simulink model "catvehicle_hoffmannFollower"  (R2016a)
settings: Solver=FixedStepAuto  StartTime=0.0  StopTime=inf  FixedStep=0.05  RelTol=1e-3
undefined symbols (not defined in the file or in its folder): Angular, Linear, Pose
libraries: robotlib x5, aerolibtransform2 x2
settings Model: Creator=sprinkle  LastModifiedBy=sprinkle
settings DataIOCC: LimitDataPoints=on
settings OptimizationCC: OptimizeModelRefInitCode=on  LifeSpan=Inf  MaxStackSize=64
settings DebuggingCC: AllowSymbolicDim=off
settings HardwareCC: ProdBitPerPointer=32  ProdLargestAtomicFloat=None  ProdIntDivRoundTo=Undefined  ProdEndianess=Unspecified  ProdWordSize=32  ProdHWDeviceType=Generic->Unspecified (assume 32-bit Generic)
settings ModelReferenceCC: PropagateSignalLabelsOutOfModel=off
settings RTWCC: SystemTargetFile=ert.tlc  HardwareBoard=Robot Operating System (ROS)  TemplateMakefile=ert_default_tmf  GenerateReport=on  Toolchain=Catkin  BuildConfiguration=Faster Runs  IncludeHyperlinkInReport=on  LaunchReport=on  TargetLang=C++  GenerateTraceInfo=on  GenerateTraceReport=on  GenerateTraceReportSl=on  GenerateTraceReportSf=on  GenerateTraceReportEml=on
settings CodeAppCC: ForceParamTrailComments=on  IgnoreCustomStorageClasses=off  OperatorAnnotations=on  SimulinkDataObjDesc=on  SFDataObjDesc=on  MATLABFcnDesc=on  InsertBlockDesc=on  MATLABSourceComments=on

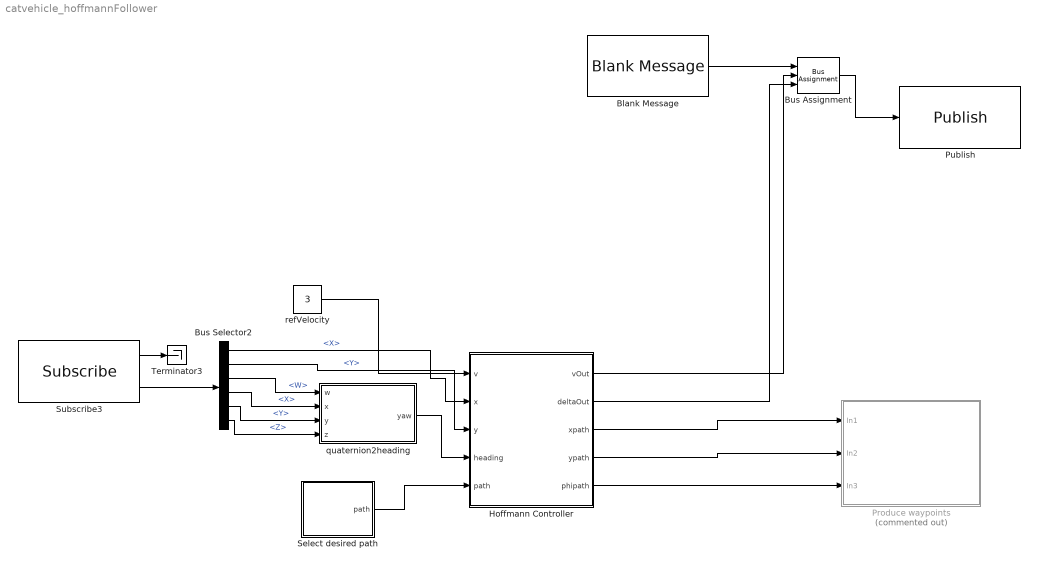
== system catvehicle_hoffmannFollower ==
  Blank Message : robotlib/Blank Message  SourceLibraryInfo=This block requires Robotics System Toolbox  messageType=geometry_msgs/Twist  SampleTime=inf
  Bus Assignment : BusAssignment  AssignedSignals=Linear.X,Angular.Z
  Bus Selector2 : BusSelector  OutputSignals=Pose.Pose.Position.X,Pose.Pose.Position.Y,Pose.Pose.Orientation.W,Pose.Pose.Orientation.X,Pose.Pose.Orientation.Y,Pose.Pose.Orientation.Z
  Hoffmann Controller : Subsystem
  Produce waypoints : Subsystem  Commented=on
  Publish : robotlib/Publish  SourceLibraryInfo=This block requires Robotics System Toolbox  topicSource=Specify your own  topic=/catvehicle/cmd_vel  messageType=geometry_msgs/Twist  messageQueueLength=1
  Select desired path : Subsystem
  Subscribe3 : robotlib/Subscribe  SourceLibraryInfo=This block requires Robotics System Toolbox  topicSource=Specify your own  topic=/catvehicle/odom  messageType=nav_msgs/Odometry  sampleTime=-1  messageQueueLength=1
  Terminator3 : Terminator
  quaternion2heading : Subsystem
  refVelocity : Constant  Value=3
  wires:
  Blank Message/1 -> Bus Assignment/1
  Bus Assignment/1 -> Publish/1
  Subscribe3/1 -> Terminator3/1
  Subscribe3/2 -> Bus Selector2/1
  refVelocity/1 -> Hoffmann Controller/1(v)
  Bus Selector2/1 -> Hoffmann Controller/2(x)  "<X>"
  Bus Selector2/2 -> Hoffmann Controller/3(y)  "<Y>"
  Hoffmann Controller/2(deltaOut) -> Bus Assignment/3
  Select desired path/1(path) -> Hoffmann Controller/5(path)
  quaternion2heading/1(yaw) -> Hoffmann Controller/4(heading)
  Bus Selector2/3 -> quaternion2heading/1(w)  "<W>"
  Bus Selector2/4 -> quaternion2heading/2(x)  "<X>"
  Bus Selector2/5 -> quaternion2heading/3(y)  "<Y>"
  Bus Selector2/6 -> quaternion2heading/4(z)  "<Z>"
  Hoffmann Controller/1(vOut) -> Bus Assignment/2
  Hoffmann Controller/3(xpath) -> Produce waypoints/1(In1)
  Hoffmann Controller/4(ypath) -> Produce waypoints/2(In2)
  Hoffmann Controller/5(phipath) -> Produce waypoints/3(In3)

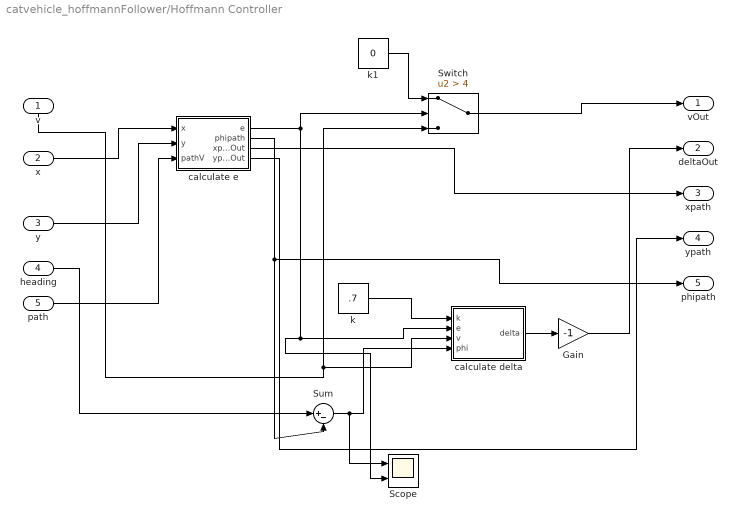
== system catvehicle_hoffmannFollower/Hoffmann Controller ==
  v : Inport
  x : Inport  Port=2
  y : Inport  Port=3
  heading : Inport  Port=4
  path : Inport  Port=5
  Gain : Gain  Gain=-1
  Scope : Scope  NumInputPorts=2
  Sum : Sum  Inputs=|+-
  Switch : Switch  Criteria=u2 > Threshold  Threshold=4
  calculate delta : MATLAB Function  TreatAsAtomicUnit=on
  calculate e : MATLAB Function  TreatAsAtomicUnit=on
  k : Constant  Value=.7
  k1 : Constant  Value=0
  vOut : Outport
  deltaOut : Outport  Port=2
  xpath : Outport  Port=3
  ypath : Outport  Port=4
  phipath : Outport  Port=5
  wires:
  v/1 -> Switch/3, calculate delta/3(v)
  path/1 -> calculate e/3(pathV)
  x/1 -> calculate e/1(x)
  y/1 -> calculate e/2(y)
  calculate e/2(phipath) -> phipath/1, Sum/2
  calculate e/1(e) -> Switch/2, Scope/2, calculate delta/2(e)
  Sum/1 -> Scope/1, calculate delta/4(phi)
  k/1 -> calculate delta/1(k)
  calculate e/3(xpathOut) -> xpath/1
  calculate e/4(ypathOut) -> ypath/1
  Switch/1 -> vOut/1
  k1/1 -> Switch/1
  heading/1 -> Sum/1
  calculate delta/1(delta) -> Gain/1
  Gain/1 -> deltaOut/1

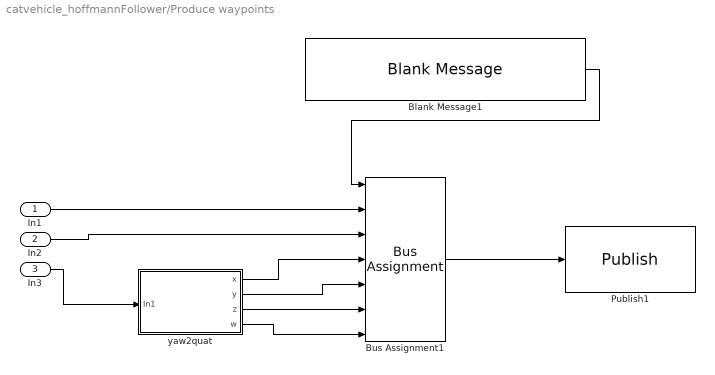
== system catvehicle_hoffmannFollower/Produce waypoints ==
  In1 : Inport
  In2 : Inport  Port=2
  In3 : Inport  Port=3
  Blank Message1 : robotlib/Blank Message  SourceLibraryInfo=This block requires Robotics System Toolbox  messageType=visualization_msgs/InteractiveMarkerPose  SampleTime=inf
  Bus Assignment1 : BusAssignment  AssignedSignals=Pose.Position.X,Pose.Position.Y,Pose.Orientation.X,Pose.Orientation.Y,Pose.Orientation.Z,Pose.Orientation.W
  Publish1 : robotlib/Publish  SourceLibraryInfo=This block requires Robotics System Toolbox  topicSource=Specify your own  topic=/catvehicle/waypoint  messageType=visualization_msgs/InteractiveMarkerPose  messageQueueLength=1
  yaw2quat : Subsystem
  wires:
  Blank Message1/1 -> Bus Assignment1/1
  Bus Assignment1/1 -> Publish1/1
  In1/1 -> Bus Assignment1/2
  In2/1 -> Bus Assignment1/3
  In3/1 -> yaw2quat/1(In1)
  yaw2quat/1(x) -> Bus Assignment1/4
  yaw2quat/2(y) -> Bus Assignment1/5
  yaw2quat/3(z) -> Bus Assignment1/6
  yaw2quat/4(w) -> Bus Assignment1/7

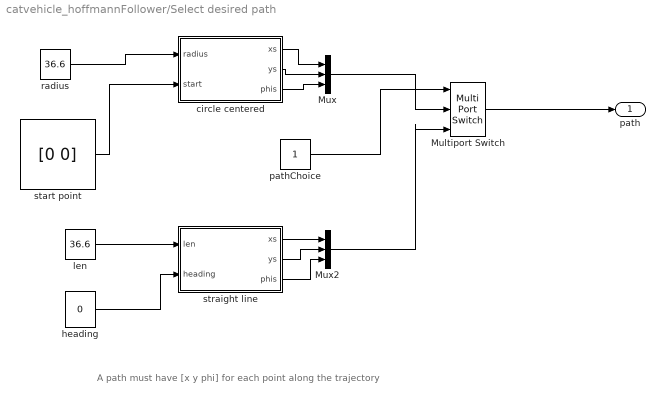
== system catvehicle_hoffmannFollower/Select desired path ==
  note: A path must have [x y phi] for each point along the trajectory
  Multiport Switch : MultiPortSwitch  Inputs=2
  Mux : Mux  Inputs=3
  Mux2 : Mux  Inputs=3
  circle centered : MATLAB Function  TreatAsAtomicUnit=on
  heading : Constant  Value=0
  len : Constant  Value=36.6
  "pathChoice " : Constant
  radius : Constant  Value=36.6
  start point : Constant  Value=[0 0]
  straight line : MATLAB Function  TreatAsAtomicUnit=on
  path : Outport
  wires:
  radius/1 -> circle centered/1(radius)
  start point/1 -> circle centered/2(start)
  "pathChoice "/1 -> Multiport Switch/1
  circle centered/2(ys) -> Mux/2
  circle centered/1(xs) -> Mux/1
  Multiport Switch/1 -> path/1
  len/1 -> straight line/1(len)
  heading/1 -> straight line/2(heading)
  straight line/1(xs) -> Mux2/1
  straight line/2(ys) -> Mux2/2
  Mux2/1 -> Multiport Switch/3
  Mux/1 -> Multiport Switch/2
  straight line/3(phis) -> Mux2/3
  circle centered/3(phis) -> Mux/3

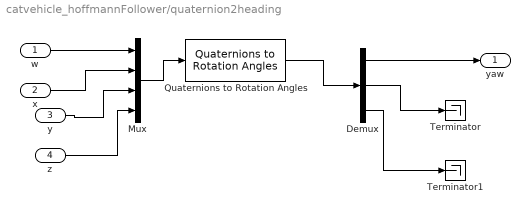
== system catvehicle_hoffmannFollower/quaternion2heading ==
  w : Inport
  x : Inport  Port=2
  y : Inport  Port=3
  z : Inport  Port=4
  Demux : Demux  Outputs=3
  Mux : Mux
  Quaternions to Rotation Angles : aerolibtransform2/Quaternions to Rotation Angles  rotationOrder=ZYX
  Terminator : Terminator
  Terminator1 : Terminator
  yaw : Outport
  wires:
  Quaternions to Rotation Angles/1 -> Demux/1
  Demux/2 -> Terminator/1
  Demux/3 -> Terminator1/1
  Demux/1 -> yaw/1
  w/1 -> Mux/1
  x/1 -> Mux/2
  y/1 -> Mux/3
  z/1 -> Mux/4
  Mux/1 -> Quaternions to Rotation Angles/1

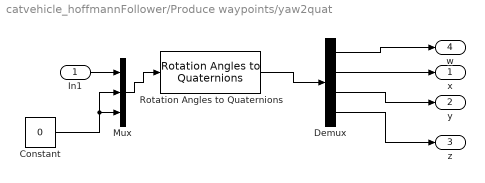
== system catvehicle_hoffmannFollower/Produce waypoints/yaw2quat ==
  In1 : Inport
  Constant : Constant  Value=0
  Demux : Demux
  Mux : Mux  Inputs=3
  Rotation Angles to Quaternions : aerolibtransform2/Rotation Angles to Quaternions  rotationOrder=ZYX
  x : Outport
  y : Outport  Port=2
  z : Outport  Port=3
  w : Outport  Port=4
  wires:
  Rotation Angles to Quaternions/1 -> Demux/1
  Demux/1 -> w/1
  Demux/2 -> x/1
  Demux/3 -> y/1
  Demux/4 -> z/1
  In1/1 -> Mux/1
  Mux/1 -> Rotation Angles to Quaternions/1
  Constant/1 -> Mux/3, Mux/2

== matlab function catvehicle_hoffmannFollower/Hoffmann Controller/calculate e ==
  data: e output; x input; y input; pathV input; phipath output; xpathOut output; ypathOut output
function [e,phipath,xpathOut,ypathOut] = fcn(x,y,pathV)
%#codegen
path=reshape(pathV,[],3);
x1 = path(1,1);
y1 = path(1,2);
phi1=path(1,3);
etmp = inf;
e = inf;
index=1;
% find the nearest x,y
for i=1:length(path)
   etmp = sqrt((x-path(i,1))^2+(y-path(i,2))^2);
   if( etmp < e )
       e = etmp;
       index=i;
   end
end

xpathOut=path(index,1);
ypathOut=path(index,2);
phipath=path(index,3);

ex1 = (path(index,1)-x);
ey1 = (path(index,2)-y);
ex2 = cos(phipath);
ey2 = sin(phipath);
sinnnn = ex1*ey2-ey1*ex2;
e = sign(sinnnn)*e;

== matlab function catvehicle_hoffmannFollower/Hoffmann Controller/calculate delta ==
  data: delta output; k input; e input; v input; phi input
function delta = fcn(k,e,v,phi)
%#codegen
if( abs(v) < eps )
    v = eps;
end

% if phi is greater than pi (or less than -pi), then 
% we normalize to between [-pi,pi]
if( phi < -pi )
    phi = phi+2*pi;
elseif( phi > pi )
    phi = phi-2*pi;
end

delta = phi + atan2(k*e,v);

== matlab function catvehicle_hoffmannFollower/Select desired path/circle centered ==
  data: xs output; radius input; start input; ys output; phis output
function [xs,ys,phis] = fcn(radius,start)
%#codegen
angles=linspace(-pi,pi,301);
r = radius*exp(angles*1j);
xs = real(r)-radius+start(1);
ys = imag(r)+start(2);
phis=(pi/2)+angles;

% % To visualize the angles, run this code:
% radius=3.6; start=[0 0];
% angles=linspace(-pi,pi,300);
% r = radius*exp(angles*1j);
% xs = real(r)-radius+start(1);
% ys = imag(r)+start(2);
% % since the direction of travel is in the 'x' direction, the 
% % heading (phi) matchines the angle of the circle
% phis=(pi/2)+angles;
% xends=cos(phis);yends=sin(phis);
% figure;plot(xs,ys);hold on; quiver(xs,ys,xends,yends);axis equal;hold off

== matlab function catvehicle_hoffmannFollower/Select desired path/straight line ==
  data: xs output; len input; heading input; ys output; phis output
function [xs,ys,phis] = fcn(len,heading)
%#codegen
r = linspace(0,len,301);
xs = r*cos(heading);
ys = r*sin(heading);
phis = heading*ones(1,length(r));
